simulink model "AWD_Test_ABS_PID"  (Simulink 7.7)
settings: Solver=ode3  StartTime=0.0  StopTime=10  FixedStep=0.001  RelTol=1e-3
undefined symbols (not defined in the file): Bx, By, Cx, Cy, dfilt, Dx, Dy, Ex, Ey, fdesignblkfcn, g, gcbh, hg, Jw, Jz, Lf, Lr, Lw, m, r0, Rw, rx1, rx2, ry1, ry2, T_Avail, Vx0, Vy0, wRL0
libraries: simulink x6, fuzblock x5, dsparch4 x1
settings Model: Creator=ETLAB  LastModifiedBy=Kenny Schmutz
settings DebuggingCC: InheritedTsInSrcMsg=none  FcnCallInpInsideContextMsg=Enable All

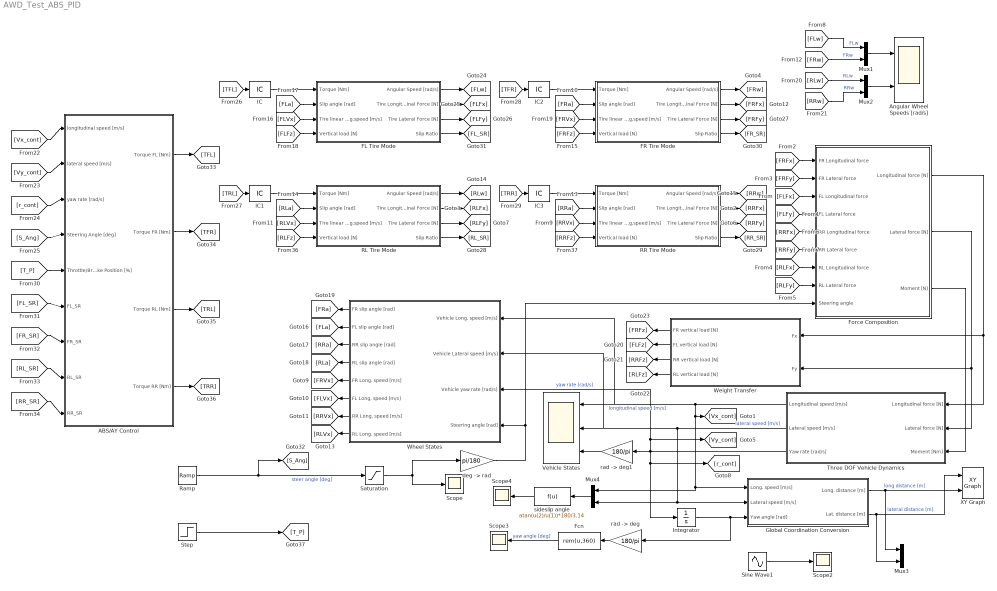
== system AWD_Test_ABS_PID ==
  ABS/AY Control : Subsystem
  Angular Wheel Speeds [rad/s] : Scope  NumInputPorts=2
      settings: YMin=-110~-110  YMax=30~30  SaveName=ScopeData7
  FL Tire Mode : Subsystem
      mask Display:
      | image(imread('Tire.bmp'),'center')
      | port_label('input', 1, 'Torque [Nm]')
      | port_label('input', 2, 'Slip angle [rad]')
      | port_label('input', 3, 'Long. speed [m/s]')
      | port_label('input', 4, 'Vertical load [N]')
      | port_label('output', 1, 'Angular speed [rad/s]')
      | port_label('output', 2, 'Long. force [N]')
      | port_label('output', 3, 'Lateral force [N]')
      | port_label('output', 4, 'Slip Ratio')
  FR Tire Mode : Subsystem
      mask Display:
      | image(imread('Tire.bmp'),'center')
      | port_label('input', 1, 'Torque [Nm]')
      | port_label('input', 2, 'Slip angle [rad]')
      | port_label('input', 3, 'Long. speed [m/s]')
      | port_label('input', 4, 'Vertical load [N]')
      | port_label('output', 1, 'Angular speed [rad/s]')
      | port_label('output', 2, 'Long. force [N]')
      | port_label('output', 3, 'Lateral force [N]')
      | port_label('output', 4, 'Slip Ratio')
  Fcn : Fcn  Expr=rem(u,360)
  Force Composition : Subsystem
  Global Coordination Conversion : Subsystem
  IC{,1..3} (4 alike) : InitialCondition  Value=0
  Integrator : Integrator
  Mux{1..4} (4 alike) : Mux  Inputs=2
  RL Tire Mode : Subsystem
      mask Display:
      | image(imread('Tire.bmp'),'center')
      | port_label('input', 1, 'Torque [Nm]')
      | port_label('input', 2, 'Slip angle [rad]')
      | port_label('input', 3, 'Long. speed [m/s]')
      | port_label('input', 4, 'Vertical load [N]')
      | port_label('output', 1, 'Angular speed [rad/s]')
      | port_label('output', 2, 'Long. force [N]')
      | port_label('output', 3, 'Lateral force [N]')
      | port_label('output', 4, 'Slip Ratio')
  RR Tire Mode : Subsystem
      mask Display:
      | image(imread('Tire.bmp'),'center')
      | port_label('input', 1, 'Torque [Nm]')
      | port_label('input', 2, 'Slip angle [rad]')
      | port_label('input', 3, 'Long. speed [m/s]')
      | port_label('input', 4, 'Vertical load [N]')
      | port_label('output', 1, 'Angular speed [rad/s]')
      | port_label('output', 2, 'Long. force [N]')
      | port_label('output', 3, 'Lateral force [N]')
  Ramp : simulink/Sources/Ramp  SystemSampleTime=-1  slope=0  start=0  X0=0
  Saturation : Saturate  UpperLimit=10  LowerLimit=-10
  Scope{,2..4} (4 alike) : Scope
      Scope settings: YMin=0.93  YMax=1
      Scope2 settings: YMin=0.525  YMax=0.825  SaveName=ScopeData3
      Scope3 settings: SaveName=ScopeData5
      Scope4 settings: YMin=0.0025  YMax=0.05  SaveName=ScopeData20
  Sine Wave1 : Sin  Frequency=0.5  SampleTime=0
  Step : Step  Time=.5  SampleTime=0
  Three DOF Vehicle Dynamics : Subsystem
      mask Display:
      | image(imread('Vehicle.bmp'),'center')
      | port_label('input', 1, 'Longitudinal force [N]')
      | port_label('input', 2, 'Lateral force [N]')
      | port_label('input', 3, 'Moment [Nm]')
      | port_label('output', 1, 'Longitudinal speed [m/s]')
      | port_label('output', 2, 'Lateral speed [m/s]')
      | port_label('output', 3, 'Yaw rate [rad/s]')
  Vehicle States : Scope  NumInputPorts=3
      settings: TimeRange=10  YMin=19.45~3.5e-033~-8.5e-032  YMax=19.56~4.4e-033~-1.5e-032  SaveName=StatesOutpus1
  Weight Transfer : Subsystem
  Wheel States : Subsystem
  XY Graph : simulink/Sinks/XY Graph  SystemSampleTime=-1  xmin=-500  xmax=500  ymin=-500  ymax=500  st=-1
  "deg -> rad" : Gain  Gain=pi/180
  "rad -> deg" : Gain  Gain=180/pi
  "rad -> deg1" : Gain  Gain=180/pi
  sideslip angle : Fcn  Expr=atan(u(2)/u(1))*180/3.14
  wires:
  RL Tire Mode/2(Tire Longitudinal Force [N]) -> [RLFx]
  RL Tire Mode/1(Angular Speed [rad/s]) -> [RLw]
  [RLVx] -> RL Tire Mode/3(Tire linear Long.speed [m/s])
  Wheel States/5(FR Long. speed [m/s]) -> [FRVx]
  Wheel States/6(FL Long. speed [m/s]) -> [FLVx]
  Wheel States/7(RR Long. speed [m/s]) -> [RRVx]
  Wheel States/8(RL Long. speed [m/s]) -> [RLVx]
  Three DOF Vehicle Dynamics/3(Yaw rate [rad/s]) -> "rad -> deg1"/1, Wheel States/3(Vehicle yaw rate [rad/s]), [Vy_cont], Integrator/1, [r_cont]  "yaw rate [rad/s]"
  Three DOF Vehicle Dynamics/2(Lateral speed [m/s]) -> Wheel States/2(Vehicle Lateral speed [m/s]), Global Coordination Conversion/2(Lateral speed [m/s]), Mux4/2, Vehicle States/2  "lateral speed [m/s]"
  Three DOF Vehicle Dynamics/1(Longitudinal speed [m/s]) -> Wheel States/1(Vehicle Long. speed [m/s]), Vehicle States/1, Global Coordination Conversion/1(Long. speed [m/s]), Mux4/1, [Vx_cont]  "longitudinal speed [m/s]"
  Wheel States/1("FR slip angle [rad] ") -> [FRa]
  Wheel States/2("FL slip angle [rad] ") -> [FLa]
  Wheel States/3("RR slip angle [rad] ") -> [RRa]
  Wheel States/4("RL slip angle [rad] ") -> [RLa]
  [RLa] -> RL Tire Mode/2(Slip angle [rad])
  Force Composition/1(Longitudinal force [N]) -> Weight Transfer/1(Fx), Three DOF Vehicle Dynamics/1(Longitudinal force [N])
  [FRFx] -> Force Composition/1(FR Longitudinal force)
  [FRFy] -> Force Composition/2(FR Lateral force)
  [FLFx] -> Force Composition/3(FL Longitudinal force)
  [FLFy] -> Force Composition/4(FL Lateral force)
  [RRFx] -> Force Composition/5(RR Longitudinal force)
  [RRFy] -> Force Composition/6(RR Lateral force)
  [RLFx] -> Force Composition/7(RL Longitudinal force)
  [RLFy] -> Force Composition/8(RL Lateral force)
  "deg -> rad"/1 -> Wheel States/4(Steering angle [rad]), Force Composition/9(Steering angle)
  "rad -> deg"/1 -> Fcn/1
  Fcn/1 -> Scope3/1  "yaw angle [deg]"
  Global Coordination Conversion/1(Long. distance [m]) -> XY Graph/2, Mux3/1  "long distance [m]"
  Global Coordination Conversion/2(Lat. distance [m]) -> XY Graph/1, Mux3/2  "lateral distance [m]"
  Weight Transfer/1(FR vertical load [N]) -> [FRFz]
  Weight Transfer/2(FL vertical load [N]) -> [FLFz]
  Weight Transfer/3(RR vertical load [N]) -> [RRFz]
  Weight Transfer/4(RL vertical load [N]) -> [RLFz]
  [RLFz] -> RL Tire Mode/4(Vertical load [N])
  Force Composition/2(Lateral force [N]) -> Weight Transfer/2(Fy), Three DOF Vehicle Dynamics/2(Lateral force [N])
  Integrator/1 -> Global Coordination Conversion/3(Yaw angle [rad]), "rad -> deg"/1
  RL Tire Mode/3(Tire Lateral Force [N]) -> [RLFy]
  [RRa] -> RR Tire Mode/2(Slip angle [rad])
  [RRVx] -> RR Tire Mode/3(Tire linear Long.speed [m/s])
  [RRFz] -> RR Tire Mode/4(Vertical load [N])
  RR Tire Mode/1(Angular Speed [rad/s]) -> [RRw]
  RR Tire Mode/2(Tire Longitudinal Force [N]) -> [RRFx]
  RR Tire Mode/3(Tire Lateral Force [N]) -> [RRFy]
  Force Composition/3(Moment [N]) -> Three DOF Vehicle Dynamics/3(Moment [Nm])
  "rad -> deg1"/1 -> Vehicle States/3
  Mux4/1 -> sideslip angle/1
  sideslip angle/1 -> Scope4/1
  Ramp/1 -> Saturation/1, [S_Ang]  "steer angle [deg]"
  Sine Wave1/1 -> Scope2/1
  FL Tire Mode/2(Tire Longitudinal Force [N]) -> [FLFx]
  FL Tire Mode/1(Angular Speed [rad/s]) -> [FLw]
  [FLVx] -> FL Tire Mode/3(Tire linear Long.speed [m/s])
  IC/1 -> FL Tire Mode/1(Torque [Nm])
  [FLa] -> FL Tire Mode/2(Slip angle [rad])
  [FLFz] -> FL Tire Mode/4(Vertical load [N])
  FL Tire Mode/3(Tire Lateral Force [N]) -> [FLFy]
  [FRa] -> FR Tire Mode/2(Slip angle [rad])
  [FRVx] -> FR Tire Mode/3(Tire linear Long.speed [m/s])
  [FRFz] -> FR Tire Mode/4(Vertical load [N])
  FR Tire Mode/1(Angular Speed [rad/s]) -> [FRw]
  FR Tire Mode/2(Tire Longitudinal Force [N]) -> [FRFx]
  FR Tire Mode/3(Tire Lateral Force [N]) -> [FRFy]
  Saturation/1 -> "deg -> rad"/1, Scope/1
  [FLw] -> Mux1/1  "FLw"
  [FRw] -> Mux1/2  "FRw"
  [RLw] -> Mux2/1  "RLw"
  [RRw] -> Mux2/2  "RRw"
  Mux1/1 -> Angular Wheel Speeds [rad/s]/1
  Mux2/1 -> Angular Wheel Speeds [rad/s]/2
  [Vx_cont] -> ABS/AY Control/1(longitudinal speed [m/s])
  [Vy_cont] -> ABS/AY Control/2(lateral speed [m/s])
  [r_cont] -> ABS/AY Control/3(yaw rate [rad/s])
  RL Tire Mode/4("Slip Ratio ") -> [RL_SR]
  RR Tire Mode/4(Slip Ratio) -> [RR_SR]
  FR Tire Mode/4(Slip Ratio) -> [FR_SR]
  FL Tire Mode/4(Slip Ratio) -> [FL_SR]
  [S_Ang] -> ABS/AY Control/4(Steering Angle [deg])
  [TFL] -> IC/1
  IC1/1 -> RL Tire Mode/1(Torque [Nm])
  [TRL] -> IC1/1
  IC2/1 -> FR Tire Mode/1(Torque [Nm])
  [TFR] -> IC2/1
  IC3/1 -> RR Tire Mode/1(Torque [Nm])
  [TRR] -> IC3/1
  ABS/AY Control/1(Torque FL [Nm]) -> [TFL]
  ABS/AY Control/2(Torque FR [Nm]) -> [TFR]
  ABS/AY Control/3(Torque RL [Nm]) -> [TRL]
  ABS/AY Control/4(Torque RR [Nm]) -> [TRR]
  [T_P] -> ABS/AY Control/5(Throttle/Brake Position [%])
  [FL_SR] -> ABS/AY Control/6(FL_SR)
  [FR_SR] -> ABS/AY Control/7(FR_SR)
  [RL_SR] -> ABS/AY Control/8(RL_SR)
  [RR_SR] -> ABS/AY Control/9(RR_SR)
  Step/1 -> [T_P]

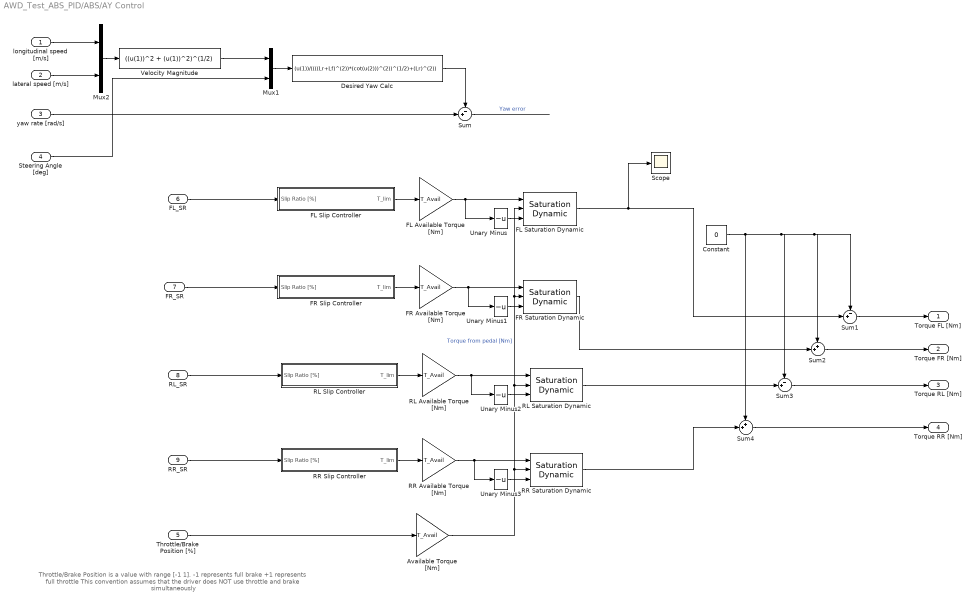
== system AWD_Test_ABS_PID/ABS/AY Control ==
  note: Throttle/Brake Position is a value with range [-1 1].
      | -1 represents full brake
      | +1 represents full throttle
      | This convention assumes that the driver does NOT use throttle and brake simultaneously
  longitudinal speed [m/s] : Inport
  lateral speed [m/s] : Inport  Port=2
  yaw rate [rad/s] : Inport  Port=3
  Steering Angle [deg] : Inport  Port=4
  Throttle/Brake Position [%] : Inport  Port=5
  FL_SR : Inport  Port=6
  FR_SR : Inport  Port=7
  RL_SR : Inport  Port=8
  RR_SR : Inport  Port=9
  Available Torque [Nm] : Gain  Gain=T_Avail
  Constant : Constant  Value=0
  Desired Yaw Calc : Fcn  Expr=(u(1))/((((Lr+Lf)^(2))*(cot(u(2)))^(2))^(1/2)+(Lr)^(2))
  FL Available Torque [Nm] : Gain  Gain=T_Avail
  FL Saturation Dynamic : simulink/Discontinuities/Saturation Dynamic  SystemSampleTime=-1  OutMin=[]  OutMax=[]  OutDataTypeStr=Inherit: Same as second input  OutDataType=fixdt(1, 16)  OutScaling=2^-10  DoSatur=off
  FL Slip Controller : Subsystem
  FR Available Torque [Nm] : Gain  Gain=T_Avail
  FR Saturation Dynamic : simulink/Discontinuities/Saturation Dynamic  SystemSampleTime=-1  OutMin=[]  OutMax=[]  OutDataTypeStr=Inherit: Same as second input  OutDataType=fixdt(1, 16)  OutScaling=2^-10  DoSatur=off
  FR Slip Controller : Subsystem
  Mux1 : Mux  Inputs=2
  Mux2 : Mux  Inputs=2
  RL Available Torque [Nm] : Gain  Gain=T_Avail
  RL Saturation Dynamic : simulink/Discontinuities/Saturation Dynamic  SystemSampleTime=-1  OutMin=[]  OutMax=[]  OutDataTypeStr=Inherit: Same as second input  OutDataType=fixdt(1, 16)  OutScaling=2^-10  DoSatur=off
  RL Slip Controller : Subsystem
  RR Available Torque [Nm] : Gain  Gain=T_Avail
  RR Saturation Dynamic : simulink/Discontinuities/Saturation Dynamic  SystemSampleTime=-1  OutMin=[]  OutMax=[]  OutDataTypeStr=Inherit: Same as second input  OutDataType=fixdt(1, 16)  OutScaling=2^-10  DoSatur=off
  RR Slip Controller : Subsystem
  Scope : Scope
      settings: YMin=-93.5444  YMax=-84.6354  SaveName=ScopeData9
  Sum : Sum  Inputs=-+|
  Sum1 : Sum  Inputs=-+|
  Sum2 : Sum  Inputs=++|
  Sum3 : Sum  Inputs=-+|
  Sum4 : Sum  Inputs=++|
  Unary Minus{,1..3} (4 alike) : UnaryMinus
  Velocity Magnitude : Fcn  Expr=((u(1))^2 + (u(1))^2)^(1/2)
  Torque FL [Nm] : Outport
  Torque FR [Nm] : Outport  Port=2
  Torque RL [Nm] : Outport  Port=3
  Torque RR [Nm] : Outport  Port=4
  wires:
  Mux1/1 -> Desired Yaw Calc/1
  lateral speed [m/s]/1 -> Mux2/2
  longitudinal speed [m/s]/1 -> Mux2/1
  Mux2/1 -> Velocity Magnitude/1
  Velocity Magnitude/1 -> Mux1/1
  Steering Angle [deg]/1 -> Mux1/2
  yaw rate [rad/s]/1 -> Sum/2
  Desired Yaw Calc/1 -> Sum/1
  Sum/1 -> ?  "Yaw error"
  Sum1/1 -> Torque FL [Nm]/1
  Sum2/1 -> Torque FR [Nm]/1
  Sum3/1 -> Torque RL [Nm]/1
  Sum4/1 -> Torque RR [Nm]/1
  Throttle/Brake Position [%]/1 -> Available Torque [Nm]/1
  Available Torque [Nm]/1 -> RR Saturation Dynamic/2, RL Saturation Dynamic/2, FR Saturation Dynamic/2, FL Saturation Dynamic/2  "Torque from pedal [Nm]"
  FL_SR/1 -> FL Slip Controller/1(Slip Ratio [%])
  FR_SR/1 -> FR Slip Controller/1(Slip Ratio [%])
  RL_SR/1 -> RL Slip Controller/1(Slip Ratio [%])
  RR_SR/1 -> RR Slip Controller/1(Slip Ratio [%])
  FL Slip Controller/1(T_lim) -> FL Available Torque [Nm]/1
  FR Slip Controller/1(T_lim) -> FR Available Torque [Nm]/1
  RL Slip Controller/1(T_lim) -> RL Available Torque [Nm]/1
  RR Slip Controller/1(T_lim) -> RR Available Torque [Nm]/1
  FL Available Torque [Nm]/1 -> FL Saturation Dynamic/1, Unary Minus/1
  Unary Minus/1 -> FL Saturation Dynamic/3
  FR Available Torque [Nm]/1 -> FR Saturation Dynamic/1, Unary Minus1/1
  Unary Minus1/1 -> FR Saturation Dynamic/3
  RL Available Torque [Nm]/1 -> RL Saturation Dynamic/1, Unary Minus2/1
  RR Available Torque [Nm]/1 -> RR Saturation Dynamic/1, Unary Minus3/1
  Unary Minus2/1 -> RL Saturation Dynamic/3
  Unary Minus3/1 -> RR Saturation Dynamic/3
  RR Saturation Dynamic/1 -> Sum4/2
  RL Saturation Dynamic/1 -> Sum3/2
  FR Saturation Dynamic/1 -> Sum2/2
  FL Saturation Dynamic/1 -> Sum1/2, Scope/1
  Constant/1 -> Sum4/1, Sum3/1, Sum1/1, Sum2/1

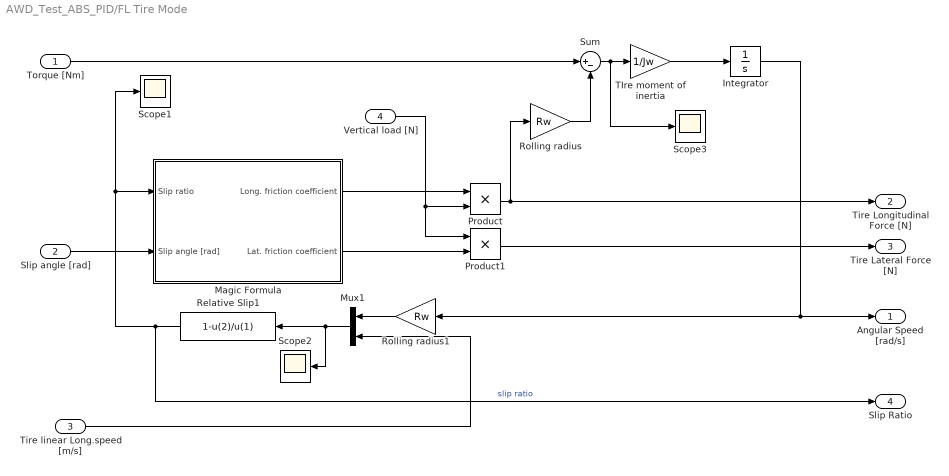
== system AWD_Test_ABS_PID/FL Tire Mode ==
  Torque [Nm] : Inport
  Slip angle [rad] : Inport  Port=2
  Tire linear Long.speed [m/s] : Inport  Port=3
  Vertical load [N] : Inport  Port=4
  Integrator : Integrator  InitialCondition=wRL0
  Magic Formula : Subsystem
      mask Type: Magic Formula (Combined Slip)
      mask Display:
      | image(imread('Magic formula.jpg'),'center')
      | port_label('input', 1, 'slip ratio')
      | port_label('input', 2, 'slip angle')
      | port_label('output', 1, 'Mux')
      | port_label('output', 2, 'Muy')
  Mux1 : Mux  Inputs=2
  Product : Product  RndMeth=Zero
  Product1 : Product  RndMeth=Zero
  Relative Slip1 : Fcn  Expr=1-u(2)/u(1)
  Rolling radius : Gain  Gain=Rw  SaturateOnIntegerOverflow=on  OutDataTypeStr=Inherit: Same as input  ParamDataTypeStr=Inherit: Same as input
  Rolling radius1 : Gain  Gain=Rw  SaturateOnIntegerOverflow=on  OutDataTypeStr=Inherit: Same as input  ParamDataTypeStr=Inherit: Same as input
  Scope1 : Scope
      settings: YMin=0.0014905  YMax=0.0014955  SaveName=ScopeData2
  Scope2 : Scope
      settings: YMin=0.001  YMax=0.013  SaveName=ScopeData11
  Scope3 : Scope
      settings: YMin=-9.46434  YMax=-9.46434  SaveName=ScopeData14
  Sum : Sum  Inputs=|+-
  TIre moment of inertia : Gain  Gain=1/Jw  SaturateOnIntegerOverflow=on  OutDataTypeStr=Inherit: Same as input  ParamDataTypeStr=Inherit: Same as input
  Angular Speed [rad/s] : Outport
  Tire Longitudinal Force [N] : Outport  Port=2
  Tire Lateral Force [N] : Outport  Port=3
  Slip Ratio : Outport  Port=4
  wires:
  Slip angle [rad]/1 -> Magic Formula/2(Slip angle [rad])
  Relative Slip1/1 -> Magic Formula/1(Slip ratio), Scope1/1, Slip Ratio/1  "slip ratio"
  Tire linear Long.speed [m/s]/1 -> Mux1/2
  Torque [Nm]/1 -> Sum/1
  Sum/1 -> TIre moment of inertia/1, Scope3/1
  TIre moment of inertia/1 -> Integrator/1
  Integrator/1 -> Angular Speed [rad/s]/1, Rolling radius1/1
  Rolling radius/1 -> Sum/2
  Mux1/1 -> Relative Slip1/1, Scope2/1
  Rolling radius1/1 -> Mux1/1
  Magic Formula/1(Long. friction coefficient) -> Product/1
  Magic Formula/2(Lat. friction coefficient) -> Product1/2
  Product/1 -> Rolling radius/1, Tire Longitudinal Force [N]/1
  Vertical load [N]/1 -> Product/2, Product1/1
  Product1/1 -> Tire Lateral Force [N]/1

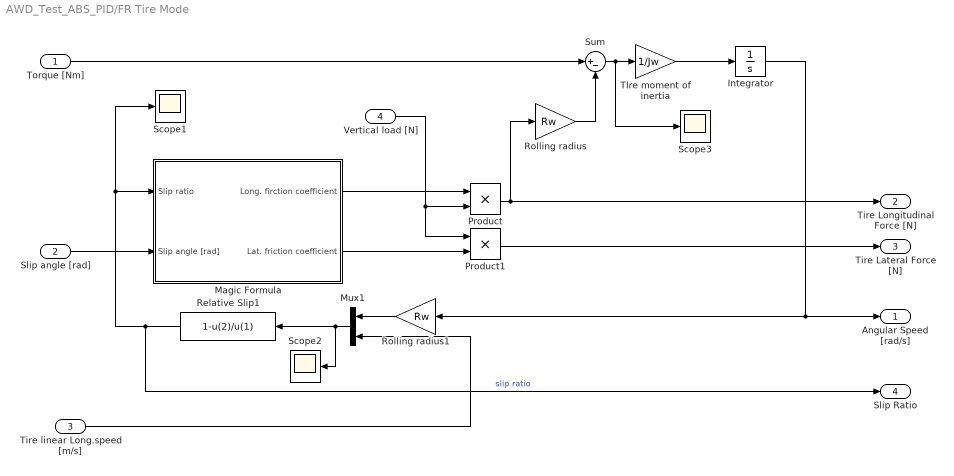
== system AWD_Test_ABS_PID/FR Tire Mode ==
  Torque [Nm] : Inport
  Slip angle [rad] : Inport  Port=2
  Tire linear Long.speed [m/s] : Inport  Port=3
  Vertical load [N] : Inport  Port=4
  Integrator : Integrator  InitialCondition=wRL0
  Magic Formula : Subsystem
      mask Type: Magic Formula (Combined Slip)
      mask Display:
      | image(imread('Magic formula.jpg'),'center')
      | port_label('input', 1, 'slip ratio')
      | port_label('input', 2, 'slip angle')
      | port_label('output', 1, 'Mux')
      | port_label('output', 2, 'Muy')
  Mux1 : Mux  Inputs=2
  Product : Product  RndMeth=Zero
  Product1 : Product  RndMeth=Zero
  Relative Slip1 : Fcn  Expr=1-u(2)/u(1)
  Rolling radius : Gain  Gain=Rw  SaturateOnIntegerOverflow=on  OutDataTypeStr=Inherit: Same as input  ParamDataTypeStr=Inherit: Same as input
  Rolling radius1 : Gain  Gain=Rw  SaturateOnIntegerOverflow=on  OutDataTypeStr=Inherit: Same as input  ParamDataTypeStr=Inherit: Same as input
  Scope1 : Scope
      settings: YMin=0.0014905  YMax=0.0014955  SaveName=ScopeData2
  Scope2 : Scope
      settings: YMin=0.001  YMax=0.013  SaveName=ScopeData11
  Scope3 : Scope
      settings: SaveName=ScopeData14
  Sum : Sum  Inputs=|+-
  TIre moment of inertia : Gain  Gain=1/Jw  SaturateOnIntegerOverflow=on  OutDataTypeStr=Inherit: Same as input  ParamDataTypeStr=Inherit: Same as input
  Angular Speed [rad/s] : Outport
  Tire Longitudinal Force [N] : Outport  Port=2
  Tire Lateral Force [N] : Outport  Port=3
  Slip Ratio : Outport  Port=4
  wires:
  Product1/1 -> Tire Lateral Force [N]/1
  Vertical load [N]/1 -> Product1/1, Product/2
  Product/1 -> Tire Longitudinal Force [N]/1, Rolling radius/1
  Magic Formula/2(Lat. friction coefficient) -> Product1/2
  Magic Formula/1(Long. firction coefficient) -> Product/1
  Rolling radius1/1 -> Mux1/1
  Mux1/1 -> Relative Slip1/1, Scope2/1
  Rolling radius/1 -> Sum/2
  Integrator/1 -> Rolling radius1/1, Angular Speed [rad/s]/1
  TIre moment of inertia/1 -> Integrator/1
  Sum/1 -> Scope3/1, TIre moment of inertia/1
  Torque [Nm]/1 -> Sum/1
  Tire linear Long.speed [m/s]/1 -> Mux1/2
  Relative Slip1/1 -> Scope1/1, Magic Formula/1(Slip ratio), Slip Ratio/1  "slip ratio"
  Slip angle [rad]/1 -> Magic Formula/2(Slip angle [rad])

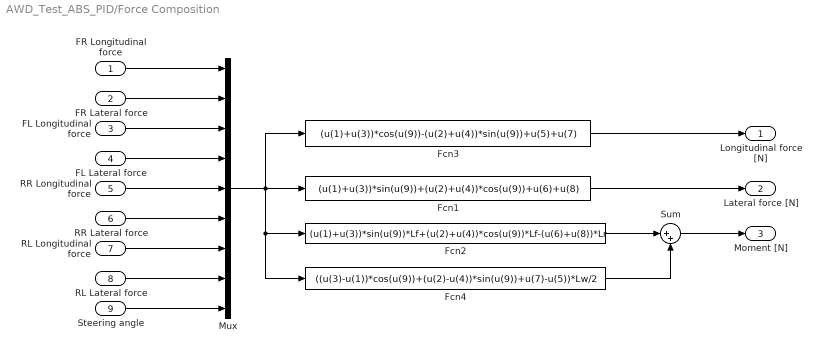
== system AWD_Test_ABS_PID/Force Composition ==
  FR Longitudinal force : Inport
  FR Lateral force : Inport  Port=2
  FL Longitudinal force : Inport  Port=3
  FL Lateral force : Inport  Port=4
  RR Longitudinal force : Inport  Port=5
  RR Lateral force : Inport  Port=6
  RL Longitudinal force : Inport  Port=7
  RL Lateral force : Inport  Port=8
  Steering angle : Inport  Port=9
  Fcn1 : Fcn  Expr=(u(1)+u(3))*sin(u(9))+(u(2)+u(4))*cos(u(9))+u(6)+u(8)
  Fcn2 : Fcn  Expr=(u(1)+u(3))*sin(u(9))*Lf+(u(2)+u(4))*cos(u(9))*Lf-(u(6)+u(8))*Lr
  Fcn3 : Fcn  Expr=(u(1)+u(3))*cos(u(9))-(u(2)+u(4))*sin(u(9))+u(5)+u(7)
  Fcn4 : Fcn  Expr=((u(3)-u(1))*cos(u(9))+(u(2)-u(4))*sin(u(9))+u(7)-u(5))*Lw/2
  Mux : Mux  Inputs=9
  Sum : Sum  Inputs=|++
  Longitudinal force [N] : Outport
  Lateral force [N] : Outport  Port=2
  Moment [N] : Outport  Port=3
  wires:
  Mux/1 -> Fcn3/1, Fcn1/1, Fcn2/1, Fcn4/1
  Fcn3/1 -> Longitudinal force [N]/1
  Fcn1/1 -> Lateral force [N]/1
  Sum/1 -> Moment [N]/1
  Fcn2/1 -> Sum/1
  Fcn4/1 -> Sum/2
  FR Longitudinal force/1 -> Mux/1
  FR Lateral force/1 -> Mux/2
  FL Longitudinal force/1 -> Mux/3
  FL Lateral force/1 -> Mux/4
  RR Longitudinal force/1 -> Mux/5
  RR Lateral force/1 -> Mux/6
  RL Longitudinal force/1 -> Mux/7
  RL Lateral force/1 -> Mux/8
  Steering angle/1 -> Mux/9

== system AWD_Test_ABS_PID/Global Coordination Conversion ==
  Long. speed [m/s] : Inport
  Lateral speed [m/s] : Inport  Port=2
  Yaw angle [rad] : Inport  Port=3
  Fcn : Fcn  Expr=cos(u(3))*u(1)-sin(u(3))*u(2)
  Fcn1 : Fcn  Expr=sin(u(3))*u(1)+cos(u(3))*u(2)
  Integrator : Integrator
  Integrator1 : Integrator
  Mux : Mux  Inputs=3
  Long. distance [m] : Outport
  Lat. distance [m] : Outport  Port=2
  wires:
  Long. speed [m/s]/1 -> Mux/1
  Lateral speed [m/s]/1 -> Mux/2
  Yaw angle [rad]/1 -> Mux/3
  Mux/1 -> Fcn/1, Fcn1/1
  Fcn/1 -> Integrator/1
  Fcn1/1 -> Integrator1/1
  Integrator/1 -> Long. distance [m]/1
  Integrator1/1 -> Lat. distance [m]/1

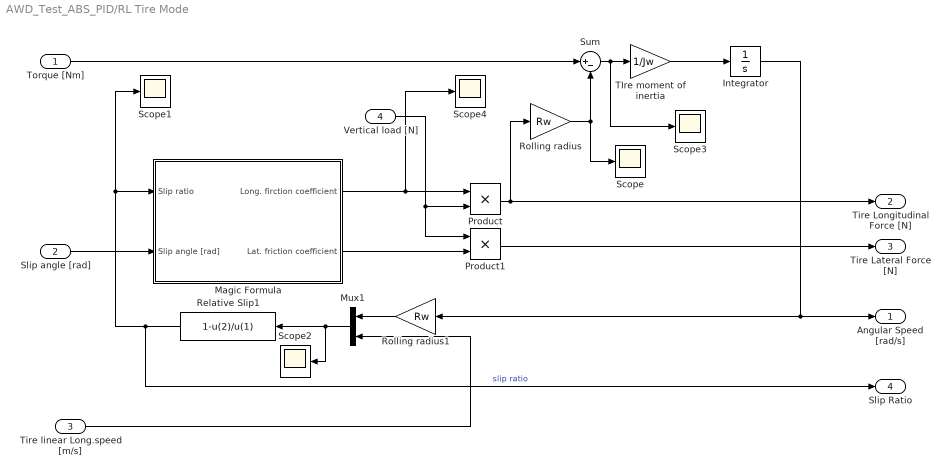
== system AWD_Test_ABS_PID/RL Tire Mode ==
  Torque [Nm] : Inport
  Slip angle [rad] : Inport  Port=2
  Tire linear Long.speed [m/s] : Inport  Port=3
  Vertical load [N] : Inport  Port=4
  Integrator : Integrator  InitialCondition=wRL0
  Magic Formula : Subsystem
      mask Type: Magic Formula (Combined Slip)
      mask Display:
      | image(imread('Magic formula.jpg'),'center')
      | port_label('input', 1, 'slip ratio')
      | port_label('input', 2, 'slip angle')
      | port_label('output', 1, 'Mux')
      | port_label('output', 2, 'Muy')
  Mux1 : Mux  Inputs=2
  Product : Product  RndMeth=Zero
  Product1 : Product  RndMeth=Zero
  Relative Slip1 : Fcn  Expr=1-u(2)/u(1)
  Rolling radius : Gain  Gain=Rw  SaturateOnIntegerOverflow=on  OutDataTypeStr=Inherit: Same as input  ParamDataTypeStr=Inherit: Same as input
  Rolling radius1 : Gain  Gain=Rw  SaturateOnIntegerOverflow=on  OutDataTypeStr=Inherit: Same as input  ParamDataTypeStr=Inherit: Same as input
  Scope{,1..4} (5 alike) : Scope
      Scope settings: SaveName=ScopeData10
      Scope1 settings: YMin=0.0014905  YMax=0.0014955  SaveName=ScopeData2
      Scope2 settings: YMin=0.001  YMax=0.013  SaveName=ScopeData11
      Scope3 settings: SaveName=ScopeData14
      Scope4 settings: SaveName=ScopeData12
  Sum : Sum  Inputs=|+-
  TIre moment of inertia : Gain  Gain=1/Jw  SaturateOnIntegerOverflow=on  OutDataTypeStr=Inherit: Same as input  ParamDataTypeStr=Inherit: Same as input
  Angular Speed [rad/s] : Outport
  Tire Longitudinal Force [N] : Outport  Port=2
  Tire Lateral Force [N] : Outport  Port=3
  "Slip Ratio " : Outport  Port=4
  wires:
  Slip angle [rad]/1 -> Magic Formula/2(Slip angle [rad])
  Relative Slip1/1 -> Magic Formula/1(Slip ratio), Scope1/1, "Slip Ratio "/1  "slip ratio"
  Tire linear Long.speed [m/s]/1 -> Mux1/2
  Torque [Nm]/1 -> Sum/1
  Sum/1 -> TIre moment of inertia/1, Scope3/1
  TIre moment of inertia/1 -> Integrator/1
  Integrator/1 -> Angular Speed [rad/s]/1, Rolling radius1/1
  Rolling radius/1 -> Sum/2, Scope/1
  Mux1/1 -> Relative Slip1/1, Scope2/1
  Rolling radius1/1 -> Mux1/1
  Magic Formula/1(Long. firction coefficient) -> Product/1, Scope4/1
  Magic Formula/2(Lat. friction coefficient) -> Product1/2
  Product/1 -> Rolling radius/1, Tire Longitudinal Force [N]/1
  Vertical load [N]/1 -> Product/2, Product1/1
  Product1/1 -> Tire Lateral Force [N]/1

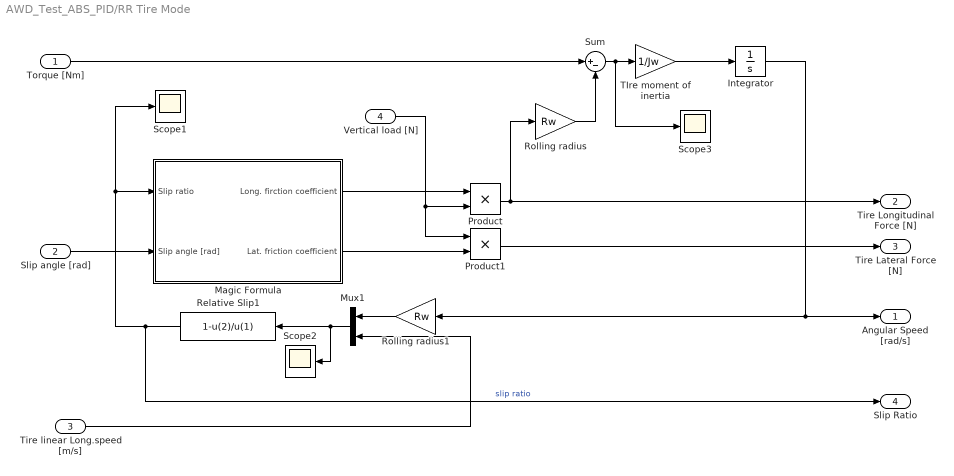
== system AWD_Test_ABS_PID/RR Tire Mode ==
  Torque [Nm] : Inport
  Slip angle [rad] : Inport  Port=2
  Tire linear Long.speed [m/s] : Inport  Port=3
  Vertical load [N] : Inport  Port=4
  Integrator : Integrator  InitialCondition=wRL0
  Magic Formula : Subsystem
      mask Type: Magic Formula (Combined Slip)
      mask Display:
      | image(imread('Magic formula.jpg'),'center')
      | port_label('input', 1, 'slip ratio')
      | port_label('input', 2, 'slip angle')
      | port_label('output', 1, 'Mux')
      | port_label('output', 2, 'Muy')
  Mux1 : Mux  Inputs=2
  Product : Product  RndMeth=Zero
  Product1 : Product  RndMeth=Zero
  Relative Slip1 : Fcn  Expr=1-u(2)/u(1)
  Rolling radius : Gain  Gain=Rw  SaturateOnIntegerOverflow=on  OutDataTypeStr=Inherit: Same as input  ParamDataTypeStr=Inherit: Same as input
  Rolling radius1 : Gain  Gain=Rw  SaturateOnIntegerOverflow=on  OutDataTypeStr=Inherit: Same as input  ParamDataTypeStr=Inherit: Same as input
  Scope1 : Scope
      settings: YMin=0.0014905  YMax=0.0014955  SaveName=ScopeData2
  Scope2 : Scope
      settings: YMin=0.001  YMax=0.013  SaveName=ScopeData11
  Scope3 : Scope
      settings: SaveName=ScopeData14
  Sum : Sum  Inputs=|+-
  TIre moment of inertia : Gain  Gain=1/Jw  SaturateOnIntegerOverflow=on  OutDataTypeStr=Inherit: Same as input  ParamDataTypeStr=Inherit: Same as input
  Angular Speed [rad/s] : Outport
  Tire Longitudinal Force [N] : Outport  Port=2
  Tire Lateral Force [N] : Outport  Port=3
  Slip Ratio : Outport  Port=4
  wires:
  Product1/1 -> Tire Lateral Force [N]/1
  Vertical load [N]/1 -> Product1/1, Product/2
  Product/1 -> Tire Longitudinal Force [N]/1, Rolling radius/1
  Magic Formula/2(Lat. friction coefficient) -> Product1/2
  Magic Formula/1(Long. firction coefficient) -> Product/1
  Rolling radius1/1 -> Mux1/1
  Mux1/1 -> Relative Slip1/1, Scope2/1
  Rolling radius/1 -> Sum/2
  Integrator/1 -> Rolling radius1/1, Angular Speed [rad/s]/1
  TIre moment of inertia/1 -> Integrator/1
  Sum/1 -> Scope3/1, TIre moment of inertia/1
  Torque [Nm]/1 -> Sum/1
  Tire linear Long.speed [m/s]/1 -> Mux1/2
  Relative Slip1/1 -> Scope1/1, Magic Formula/1(Slip ratio), Slip Ratio/1  "slip ratio"
  Slip angle [rad]/1 -> Magic Formula/2(Slip angle [rad])

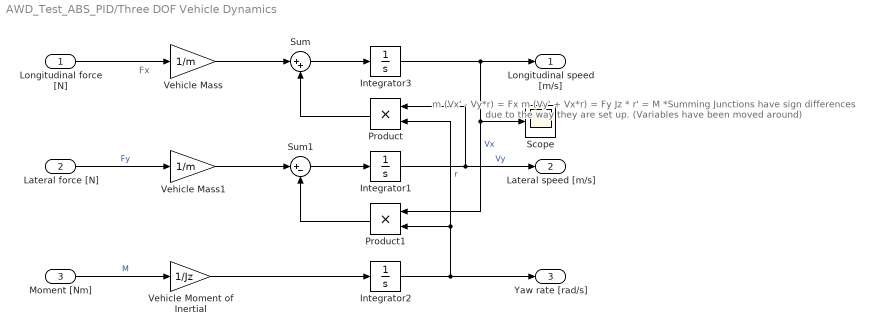
== system AWD_Test_ABS_PID/Three DOF Vehicle Dynamics ==
  note: m (Vx' - Vy*r) = Fx
      | m (Vy' + Vx*r) = Fy
      |
      | Jz * r' = M
      |
      | *Summing Junctions have sign differences due to
      | the way they are set up. (Variables have been moved around)
  note: Fx
  Longitudinal force [N] : Inport
  Lateral force [N] : Inport  Port=2
  Moment [Nm] : Inport  Port=3
  Integrator1 : Integrator  InitialCondition=Vy0  UpperSaturationLimit=1000  LowerSaturationLimit=0
  Integrator2 : Integrator  InitialCondition=r0
  Integrator3 : Integrator  InitialCondition=Vx0  UpperSaturationLimit=1000  LowerSaturationLimit=0
  Product : Product  RndMeth=Zero
  Product1 : Product  RndMeth=Zero
  Scope : Scope
      settings: SaveName=ScopeData18
  Sum : Sum  Inputs=|++
  Sum1 : Sum  Inputs=|+-
  Vehicle Mass : Gain  Gain=1/m
  Vehicle Mass1 : Gain  Gain=1/m
  Vehicle Moment of Inertial : Gain  Gain=1/Jz
  Longitudinal speed [m/s] : Outport
  Lateral speed [m/s] : Outport  Port=2
  Yaw rate [rad/s] : Outport  Port=3
  wires:
  Integrator2/1 -> Yaw rate [rad/s]/1, Product/2, Product1/2  "r"
  Moment [Nm]/1 -> Vehicle Moment of Inertial/1  "M"
  Integrator1/1 -> Product/1, Lateral speed [m/s]/1  "Vy"
  Integrator3/1 -> Longitudinal speed [m/s]/1, Product1/1, Scope/1  "Vx"
  Vehicle Moment of Inertial/1 -> Integrator2/1
  Vehicle Mass1/1 -> Sum1/1
  Lateral force [N]/1 -> Vehicle Mass1/1  "Fy"
  Vehicle Mass/1 -> Sum/1
  Sum1/1 -> Integrator1/1
  Product1/1 -> Sum1/2
  Sum/1 -> Integrator3/1
  Product/1 -> Sum/2
  Longitudinal force [N]/1 -> Vehicle Mass/1

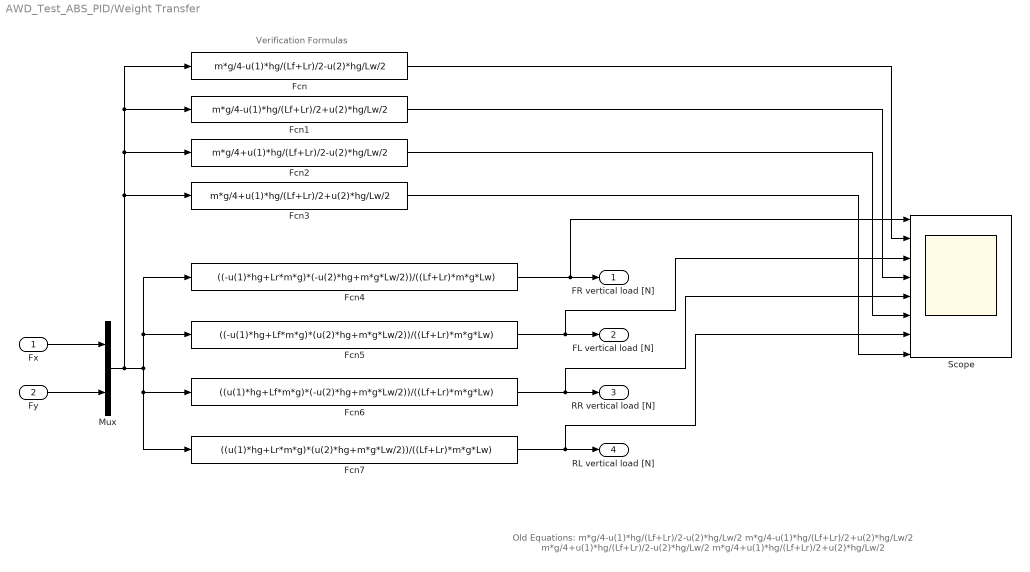
== system AWD_Test_ABS_PID/Weight Transfer ==
  note: Old Equations:
      | m*g/4-u(1)*hg/(Lf+Lr)/2-u(2)*hg/Lw/2
      | m*g/4-u(1)*hg/(Lf+Lr)/2+u(2)*hg/Lw/2
      | m*g/4+u(1)*hg/(Lf+Lr)/2-u(2)*hg/Lw/2
      | m*g/4+u(1)*hg/(Lf+Lr)/2+u(2)*hg/Lw/2
  note: Verification Formulas
  Fx : Inport
  Fy : Inport  Port=2
  Fcn : Fcn  Expr=m*g/4-u(1)*hg/(Lf+Lr)/2-u(2)*hg/Lw/2
  Fcn1 : Fcn  Expr=m*g/4-u(1)*hg/(Lf+Lr)/2+u(2)*hg/Lw/2
  Fcn2 : Fcn  Expr=m*g/4+u(1)*hg/(Lf+Lr)/2-u(2)*hg/Lw/2
  Fcn3 : Fcn  Expr=m*g/4+u(1)*hg/(Lf+Lr)/2+u(2)*hg/Lw/2
  Fcn4 : Fcn  Expr=((-u(1)*hg+Lr*m*g)*(-u(2)*hg+m*g*Lw/2))/((Lf+Lr)*m*g*Lw)
  Fcn5 : Fcn  Expr=((-u(1)*hg+Lf*m*g)*(u(2)*hg+m*g*Lw/2))/((Lf+Lr)*m*g*Lw)
  Fcn6 : Fcn  Expr=((u(1)*hg+Lf*m*g)*(-u(2)*hg+m*g*Lw/2))/((Lf+Lr)*m*g*Lw)
  Fcn7 : Fcn  Expr=((u(1)*hg+Lr*m*g)*(u(2)*hg+m*g*Lw/2))/((Lf+Lr)*m*g*Lw)
  Mux : Mux  Inputs=2
  Scope : Scope  NumInputPorts=8
      settings: TimeRange=20  YMin=0~3100~3800~4000~3100~3100~4000~4000  YMax=10000~3400~4400~4300~3400~3400~4300~4300  SaveName=ScopeData6  MaxDataPoints=21000
  FR vertical load [N] : Outport
  FL vertical load [N] : Outport  Port=2
  RR vertical load [N] : Outport  Port=3
  RL vertical load [N] : Outport  Port=4
  wires:
  Fy/1 -> Mux/2
  Fx/1 -> Mux/1
  Fcn4/1 -> FR vertical load [N]/1, Scope/1
  Fcn5/1 -> FL vertical load [N]/1, Scope/3
  Fcn6/1 -> RR vertical load [N]/1, Scope/5
  Fcn7/1 -> RL vertical load [N]/1, Scope/7
  Fcn/1 -> Scope/2
  Fcn1/1 -> Scope/4
  Fcn2/1 -> Scope/6
  Fcn3/1 -> Scope/8
  Mux/1 -> Fcn4/1, Fcn5/1, Fcn6/1, Fcn7/1, Fcn3/1, Fcn2/1, Fcn1/1, Fcn/1

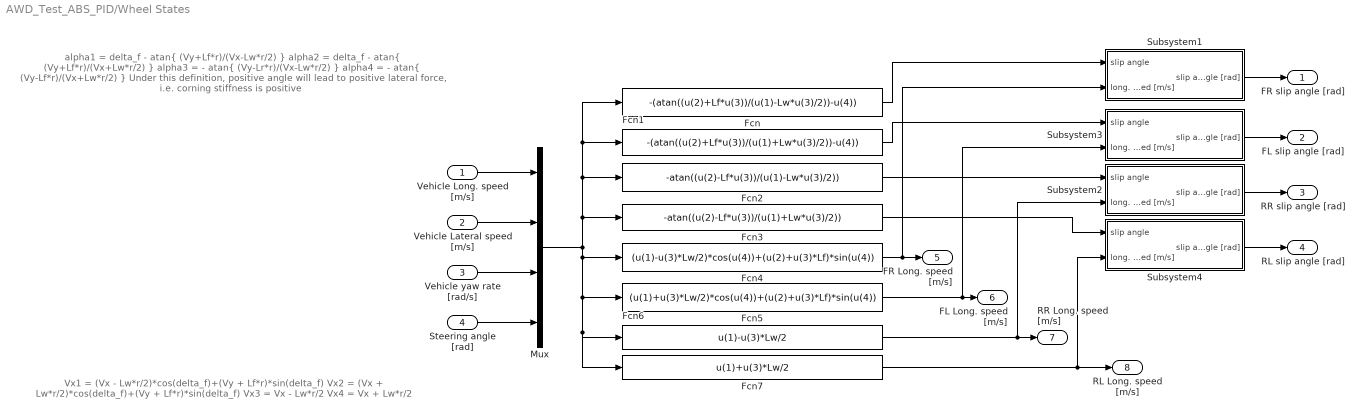
== system AWD_Test_ABS_PID/Wheel States ==
  note: alpha1 = delta_f - atan{ (Vy+Lf*r)/(Vx-Lw*r/2) }
      | alpha2 = delta_f - atan{ (Vy+Lf*r)/(Vx+Lw*r/2) }
      | alpha3 = - atan{ (Vy-Lr*r)/(Vx-Lw*r/2) }
      | alpha4 = - atan{ (Vy-Lf*r)/(Vx+Lw*r/2) }
      | Under this definition, positive angle will lead to  positive lateral force,
      | i.e. corning stiffness is positive
  note: Vx1 = (Vx - Lw*r/2)*cos(delta_f)+(Vy + Lf*r)*sin(delta_f)
      | Vx2 = (Vx + Lw*r/2)*cos(delta_f)+(Vy + Lf*r)*sin(delta_f)
      | Vx3 = Vx - Lw*r/2
      | Vx4 = Vx + Lw*r/2
  Vehicle Long. speed [m/s] : Inport
  Vehicle Lateral speed [m/s] : Inport  Port=2
  Vehicle yaw rate [rad/s] : Inport  Port=3
  Steering angle [rad] : Inport  Port=4
  Fcn : Fcn  Expr=-(atan((u(2)+Lf*u(3))/(u(1)-Lw*u(3)/2))-u(4))
  Fcn1 : Fcn  Expr=-(atan((u(2)+Lf*u(3))/(u(1)+Lw*u(3)/2))-u(4))
  Fcn2 : Fcn  Expr=-atan((u(2)-Lf*u(3))/(u(1)-Lw*u(3)/2))
  Fcn3 : Fcn  Expr=-atan((u(2)-Lf*u(3))/(u(1)+Lw*u(3)/2))
  Fcn4 : Fcn  Expr=(u(1)-u(3)*Lw/2)*cos(u(4))+(u(2)+u(3)*Lf)*sin(u(4))
  Fcn5 : Fcn  Expr=(u(1)+u(3)*Lw/2)*cos(u(4))+(u(2)+u(3)*Lf)*sin(u(4))
  Fcn6 : Fcn  Expr=u(1)-u(3)*Lw/2
  Fcn7 : Fcn  Expr=u(1)+u(3)*Lw/2
  Mux : Mux
  Subsystem1 : Subsystem
  Subsystem2 : Subsystem
  Subsystem3 : Subsystem
  Subsystem4 : Subsystem
  "FR slip angle [rad] " : Outport
  "FL slip angle [rad] " : Outport  Port=2
  "RR slip angle [rad] " : Outport  Port=3
  "RL slip angle [rad] " : Outport  Port=4
  FR Long. speed [m/s] : Outport  Port=5
  FL Long. speed [m/s] : Outport  Port=6
  RR Long. speed [m/s] : Outport  Port=7
  RL Long. speed [m/s] : Outport  Port=8
  wires:
  Vehicle yaw rate [rad/s]/1 -> Mux/3
  Vehicle Lateral speed [m/s]/1 -> Mux/2
  Vehicle Long. speed [m/s]/1 -> Mux/1
  Steering angle [rad]/1 -> Mux/4
  Fcn4/1 -> FR Long. speed [m/s]/1, Subsystem1/2(long. speed [m/s])
  Fcn5/1 -> FL Long. speed [m/s]/1, Subsystem3/2(long. speed [m/s])
  Fcn6/1 -> RR Long. speed [m/s]/1, Subsystem2/2(long. speed [m/s])
  Fcn7/1 -> RL Long. speed [m/s]/1, Subsystem4/2(long. speed [m/s])
  Mux/1 -> Fcn5/1, Fcn7/1, Fcn6/1, Fcn4/1, Fcn3/1, Fcn2/1, Fcn1/1, Fcn/1
  Subsystem1/1(slip angle [rad]) -> "FR slip angle [rad] "/1
  Fcn/1 -> Subsystem1/1(slip angle)
  Subsystem3/1(slip angle [rad]) -> "FL slip angle [rad] "/1
  Fcn1/1 -> Subsystem3/1(slip angle)
  Fcn2/1 -> Subsystem2/1(slip angle)
  Fcn3/1 -> Subsystem4/1(slip angle)
  Subsystem2/1(slip angle [rad]) -> "RR slip angle [rad] "/1
  Subsystem4/1(slip angle [rad]) -> "RL slip angle [rad] "/1

== system AWD_Test_ABS_PID/ABS/AY Control/FL Slip Controller ==
  Slip Ratio [%] : Inport
  Abs : Abs
  Derivative : Derivative
  Fuzzy Logic  Controller  with Ruleviewer : fuzblock/Fuzzy Logic  Controller  with Ruleviewer  SystemSampleTime=-1  fismatrix=Fuzzy_Slip_Controller  Ts=.1
  Lowpass Filter : Subsystem  DialogController=fdesignblkfcn  DialogControllerArgs=DataTag1  InitFcn=fdesignblkfcn(gcbh, {'InitFcn'});
      settings: CopyFcn=fdesignblkfcn(gcbh, {'CopyFcn'});
      mask Type: Lowpass Filter
      mask Description: Design a lowpass filter
      mask Help: helpview(mapfilelocation('dsp'), 'dsplowpassfilter');
      mask Display: disp('Lowpass')
  Mux1 : Mux  Inputs=2
  Scope : Scope
      settings: SaveName=ScopeData8
  Unary Minus : UnaryMinus
  Zero-Order Hold : ZeroOrderHold  SampleTime=.001
  T_lim : Outport
  wires:
  Derivative/1 -> Mux1/1
  Mux1/1 -> Fuzzy Logic  Controller  with Ruleviewer/1
  Fuzzy Logic  Controller  with Ruleviewer/1 -> Scope/1, T_lim/1
  Slip Ratio [%]/1 -> Zero-Order Hold/1
  Abs/1 -> Unary Minus/1
  Unary Minus/1 -> Mux1/2
  Lowpass Filter/1(Out) -> Derivative/1, Abs/1
  Zero-Order Hold/1 -> Lowpass Filter/1(In)

== system AWD_Test_ABS_PID/ABS/AY Control/FR Slip Controller ==
  Slip Ratio [%] : Inport
  Abs : Abs
  Derivative : Derivative
  Fuzzy Logic  Controller  with Ruleviewer : fuzblock/Fuzzy Logic  Controller  with Ruleviewer  SystemSampleTime=-1  fismatrix=Fuzzy_Slip_Controller  Ts=.1
  Mux1 : Mux  Inputs=2
  Scope : Scope
      settings: SaveName=ScopeData8
  Unary Minus : UnaryMinus
  T_lim : Outport
  wires:
  Derivative/1 -> Mux1/1
  Mux1/1 -> Fuzzy Logic  Controller  with Ruleviewer/1
  Fuzzy Logic  Controller  with Ruleviewer/1 -> Scope/1, T_lim/1
  Abs/1 -> Unary Minus/1
  Unary Minus/1 -> Mux1/2
  Slip Ratio [%]/1 -> Derivative/1, Abs/1

== system AWD_Test_ABS_PID/ABS/AY Control/RL Slip Controller ==
  Slip Ratio [%] : Inport
  Abs : Abs
  Derivative : Derivative
  Fuzzy Logic  Controller  with Ruleviewer : fuzblock/Fuzzy Logic  Controller  with Ruleviewer  SystemSampleTime=-1  fismatrix=Fuzzy_Slip_Controller  Ts=.1
  Fuzzy Logic  Controller  with Ruleviewer1 : fuzblock/Fuzzy Logic  Controller  with Ruleviewer  SystemSampleTime=-1  fismatrix=Fuzzy_Slip_Controller  Ts=.1
  Mux1 : Mux  Inputs=2
  Mux2 : Mux  Inputs=2
  Scope : Scope
      settings: SaveName=ScopeData8
  Scope1 : Scope  NumInputPorts=3
      settings: YMin=-5~-5~-5  YMax=5~5~5  SaveName=ScopeData13
  Sine Wave : Sin  Frequency=10  Phase=90  SampleTime=.01
  Sine Wave1 : Sin  Amplitude=.4  Bias=-.5  Frequency=12  SampleTime=.01
  Unary Minus : UnaryMinus
  T_lim : Outport
  wires:
  Derivative/1 -> Mux1/1
  Mux1/1 -> Fuzzy Logic  Controller  with Ruleviewer/1
  Fuzzy Logic  Controller  with Ruleviewer/1 -> Scope/1, T_lim/1
  Abs/1 -> Unary Minus/1
  Unary Minus/1 -> Mux1/2
  Slip Ratio [%]/1 -> Derivative/1, Abs/1
  Fuzzy Logic  Controller  with Ruleviewer1/1 -> Scope1/1
  Mux2/1 -> Fuzzy Logic  Controller  with Ruleviewer1/1
  Sine Wave/1 -> Mux2/1, Scope1/2
  Sine Wave1/1 -> Mux2/2, Scope1/3

== system AWD_Test_ABS_PID/ABS/AY Control/RR Slip Controller ==
  Slip Ratio [%] : Inport
  Abs : Abs
  Derivative : Derivative
  Fuzzy Logic  Controller  with Ruleviewer : fuzblock/Fuzzy Logic  Controller  with Ruleviewer  SystemSampleTime=-1  fismatrix=Fuzzy_Slip_Controller  Ts=.01
  Mux1 : Mux  Inputs=2
  Scope : Scope
      settings: SaveName=ScopeData8
  Unary Minus : UnaryMinus
  T_lim : Outport
  wires:
  Derivative/1 -> Mux1/1
  Mux1/1 -> Fuzzy Logic  Controller  with Ruleviewer/1
  Fuzzy Logic  Controller  with Ruleviewer/1 -> Scope/1, T_lim/1
  Abs/1 -> Unary Minus/1
  Unary Minus/1 -> Mux1/2
  Slip Ratio [%]/1 -> Derivative/1, Abs/1

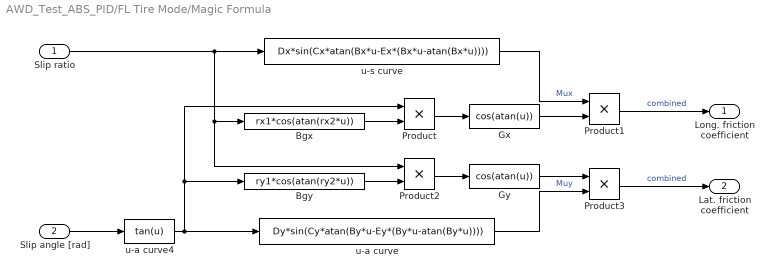
== system AWD_Test_ABS_PID/FL Tire Mode/Magic Formula ==
  Slip ratio : Inport
  Slip angle [rad] : Inport  Port=2
  Bgx : Fcn  Expr=rx1*cos(atan(rx2*u))
  Bgy : Fcn  Expr=ry1*cos(atan(ry2*u))
  Gx : Fcn  Expr=cos(atan(u))
  Gy : Fcn  Expr=cos(atan(u))
  Product{,1..3} (4 alike) : Product  RndMeth=Zero
  u-a curve : Fcn  Expr=Dy*sin(Cy*atan(By*u-Ey*(By*u-atan(By*u))))
  u-a curve4 : Fcn  Expr=tan(u)
  u-s curve : Fcn  Expr=Dx*sin(Cx*atan(Bx*u-Ex*(Bx*u-atan(Bx*u))))
  Long. friction coefficient : Outport
  Lat. friction coefficient : Outport  Port=2
  wires:
  Bgx/1 -> Product/2
  Bgy/1 -> Product2/2
  Slip angle [rad]/1 -> u-a curve4/1
  Product3/1 -> Lat. friction coefficient/1  "combined"
  Gy/1 -> Product3/1
  Product2/1 -> Gy/1
  Product1/1 -> Long. friction coefficient/1  "combined"
  Gx/1 -> Product1/2
  Product/1 -> Gx/1
  u-a curve4/1 -> Product/1, Bgy/1, u-a curve/1
  Slip ratio/1 -> Bgx/1, Product2/1, u-s curve/1
  u-a curve/1 -> Product3/2  "Muy"
  u-s curve/1 -> Product1/1  "Mux"

== system AWD_Test_ABS_PID/FR Tire Mode/Magic Formula ==
  Slip ratio : Inport
  Slip angle [rad] : Inport  Port=2
  Bgx : Fcn  Expr=rx1*cos(atan(rx2*u))
  Bgy : Fcn  Expr=ry1*cos(atan(ry2*u))
  Gx : Fcn  Expr=cos(atan(u))
  Gy : Fcn  Expr=cos(atan(u))
  Product{,1..3} (4 alike) : Product  RndMeth=Zero
  u-a curve : Fcn  Expr=Dy*sin(Cy*atan(By*u-Ey*(By*u-atan(By*u))))
  u-a curve4 : Fcn  Expr=tan(u)
  u-s curve : Fcn  Expr=Dx*sin(Cx*atan(Bx*u-Ex*(Bx*u-atan(Bx*u))))
  Long. firction coefficient : Outport
  Lat. friction coefficient : Outport  Port=2
  wires:
  u-s curve/1 -> Product1/1  "Mux"
  u-a curve/1 -> Product3/2  "Muy"
  Slip ratio/1 -> u-s curve/1, Product2/1, Bgx/1
  u-a curve4/1 -> u-a curve/1, Bgy/1, Product/1
  Product/1 -> Gx/1
  Gx/1 -> Product1/2
  Product1/1 -> Long. firction coefficient/1  "combined"
  Product2/1 -> Gy/1
  Gy/1 -> Product3/1
  Product3/1 -> Lat. friction coefficient/1  "combined"
  Slip angle [rad]/1 -> u-a curve4/1
  Bgy/1 -> Product2/2
  Bgx/1 -> Product/2

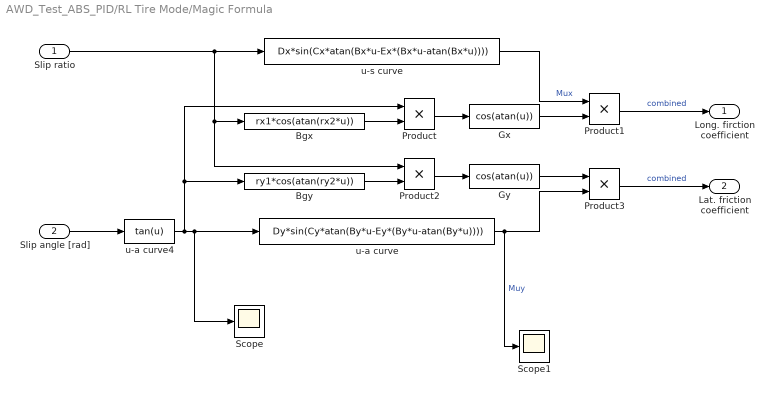
== system AWD_Test_ABS_PID/RL Tire Mode/Magic Formula ==
  Slip ratio : Inport
  Slip angle [rad] : Inport  Port=2
  Bgx : Fcn  Expr=rx1*cos(atan(rx2*u))
  Bgy : Fcn  Expr=ry1*cos(atan(ry2*u))
  Gx : Fcn  Expr=cos(atan(u))
  Gy : Fcn  Expr=cos(atan(u))
  Product{,1..3} (4 alike) : Product  RndMeth=Zero
  Scope : Scope
      settings: TimeRange=21
  Scope1 : Scope
      settings: SaveName=ScopeData4
  u-a curve : Fcn  Expr=Dy*sin(Cy*atan(By*u-Ey*(By*u-atan(By*u))))
  u-a curve4 : Fcn  Expr=tan(u)
  u-s curve : Fcn  Expr=Dx*sin(Cx*atan(Bx*u-Ex*(Bx*u-atan(Bx*u))))
  Long. firction coefficient : Outport
  Lat. friction coefficient : Outport  Port=2
  wires:
  Bgx/1 -> Product/2
  Bgy/1 -> Product2/2
  Slip angle [rad]/1 -> u-a curve4/1
  Product3/1 -> Lat. friction coefficient/1  "combined"
  Gy/1 -> Product3/1
  Product2/1 -> Gy/1
  Product1/1 -> Long. firction coefficient/1  "combined"
  Gx/1 -> Product1/2
  Product/1 -> Gx/1
  u-a curve4/1 -> Product/1, Bgy/1, u-a curve/1, Scope/1
  Slip ratio/1 -> Bgx/1, Product2/1, u-s curve/1
  u-a curve/1 -> Product3/2, Scope1/1  "Muy"
  u-s curve/1 -> Product1/1  "Mux"

== system AWD_Test_ABS_PID/RR Tire Mode/Magic Formula ==
  Slip ratio : Inport
  Slip angle [rad] : Inport  Port=2
  Bgx : Fcn  Expr=rx1*cos(atan(rx2*u))
  Bgy : Fcn  Expr=ry1*cos(atan(ry2*u))
  Gx : Fcn  Expr=cos(atan(u))
  Gy : Fcn  Expr=cos(atan(u))
  Product{,1..3} (4 alike) : Product  RndMeth=Zero
  u-a curve : Fcn  Expr=Dy*sin(Cy*atan(By*u-Ey*(By*u-atan(By*u))))
  u-a curve4 : Fcn  Expr=tan(u)
  u-s curve : Fcn  Expr=Dx*sin(Cx*atan(Bx*u-Ex*(Bx*u-atan(Bx*u))))
  Long. firction coefficient : Outport
  Lat. friction coefficient : Outport  Port=2
  wires:
  u-s curve/1 -> Product1/1  "Mux"
  u-a curve/1 -> Product3/2  "Muy"
  Slip ratio/1 -> u-s curve/1, Product2/1, Bgx/1
  u-a curve4/1 -> u-a curve/1, Bgy/1, Product/1
  Product/1 -> Gx/1
  Gx/1 -> Product1/2
  Product1/1 -> Long. firction coefficient/1  "combined"
  Product2/1 -> Gy/1
  Gy/1 -> Product3/1
  Product3/1 -> Lat. friction coefficient/1  "combined"
  Slip angle [rad]/1 -> u-a curve4/1
  Bgy/1 -> Product2/2
  Bgx/1 -> Product/2

== system AWD_Test_ABS_PID/Wheel States/Subsystem1 ==
  slip angle : Inport
  long. speed [m/s] : Inport  Port=2
  If : If
  Merge1 : Merge
  negative slip angle : Subsystem  TreatAsAtomicUnit=on
  positive slip angle : Subsystem  TreatAsAtomicUnit=on
  slip angle [rad] : Outport
  wires:
  If/2 -> negative slip angle/Action
  negative slip angle/1(-in) -> Merge1/2
  positive slip angle/1(+in) -> Merge1/1
  If/1 -> positive slip angle/Action
  long. speed [m/s]/1 -> If/1
  slip angle/1 -> negative slip angle/1(in), positive slip angle/1(in)
  Merge1/1 -> slip angle [rad]/1

== system AWD_Test_ABS_PID/Wheel States/Subsystem2 ==
  slip angle : Inport
  long. speed [m/s] : Inport  Port=2
  If : If
  Merge1 : Merge
  negative slip angle : Subsystem  TreatAsAtomicUnit=on
  positive slip angle : Subsystem  TreatAsAtomicUnit=on
  slip angle [rad] : Outport
  wires:
  Merge1/1 -> slip angle [rad]/1
  slip angle/1 -> positive slip angle/1(in), negative slip angle/1(in)
  long. speed [m/s]/1 -> If/1
  If/1 -> positive slip angle/Action
  positive slip angle/1(+in) -> Merge1/1
  negative slip angle/1(-in) -> Merge1/2
  If/2 -> negative slip angle/Action

== system AWD_Test_ABS_PID/Wheel States/Subsystem3 ==
  slip angle : Inport
  long. speed [m/s] : Inport  Port=2
  If : If
  Merge1 : Merge
  negative slip angle : Subsystem  TreatAsAtomicUnit=on
  positive slip angle : Subsystem  TreatAsAtomicUnit=on
  slip angle [rad] : Outport
  wires:
  Merge1/1 -> slip angle [rad]/1
  slip angle/1 -> positive slip angle/1(in), negative slip angle/1(in)
  long. speed [m/s]/1 -> If/1
  If/1 -> positive slip angle/Action
  positive slip angle/1(+in) -> Merge1/1
  negative slip angle/1(-in) -> Merge1/2
  If/2 -> negative slip angle/Action

== system AWD_Test_ABS_PID/Wheel States/Subsystem4 ==
  slip angle : Inport
  long. speed [m/s] : Inport  Port=2
  If : If
  Merge1 : Merge
  negative slip angle : Subsystem  TreatAsAtomicUnit=on
  positive slip angle : Subsystem  TreatAsAtomicUnit=on
  slip angle [rad] : Outport
  wires:
  If/2 -> negative slip angle/Action
  negative slip angle/1(-in) -> Merge1/2
  positive slip angle/1(+in) -> Merge1/1
  If/1 -> positive slip angle/Action
  long. speed [m/s]/1 -> If/1
  slip angle/1 -> negative slip angle/1(in), positive slip angle/1(in)
  Merge1/1 -> slip angle [rad]/1

== system AWD_Test_ABS_PID/ABS/AY Control/FL Slip Controller/Lowpass Filter ==
  In : Inport
  Generated Filter Block : dsparch4/Digital Filter  Tag=BlockMethodSubSystem  TypePopup=FIR (all zeros)  IIRFiltStruct=Direct form II transposed  AllPoleFiltStruct=Direct form  FIRFiltStruct=Direct form  CoeffSource=Specify via dialog  NumCoeffs=[0.0174383341854297 -0.00191782029741124 0.00198412368845642 -0.00202320724480635 0.00203368000831878 -0.00201284299964119 0.0019583382808233 -0.00186738997518325 0.00173746587339042 -0.0015681629128845 0.00135498370854467 -0.00110302068622745 0.000800701191448522 -0.000457496942976669 6.66695446854202e-005 0.000372926543227212 -0.000859609238705387 0.00139275199781003 -0.00197359205968968 0.00260213773222492 -0.00327367392723359 0.00399185205153304 -0.00474687033612613 0.00553984252048373 -0.00636388746973452 0.00721789141475684 -0.00809980835965676 0.00900839900993329 -0.00994311352927216 0.0109001841792156 -0.0118658172469424 0.0127965798493482 -0.0137852818010553 0.014742027667021 -0.0156964264578652 0.0166370406414232 -0.0175588861083261 0.0184562272582075 -0.0193239272144743 0.0201573063619979 -0.0209504538297715 0.0217022550324855 -0.0223968347980343 0.0230523485789057 -0.023639833722988 0.0241679591776366 -0.0246360803373166 0.025038665505458 -0.0253705205926199 0.0256294834812449 -0.0258148349606314 0.0259242151526749 0.974037626336816 0.0259242151526749 -0.0258148349606314 0.0256294834812449 -0.0253705205926199 0.025038665505458 -0.0246360803373166 0.0241679591776366 -0.023639833722988 0.0230523485789057 -0.0223968347980343 0.0217022550324855 -0.0209504538297715 0.0201573063619979 -0.0193239272144743 0.0184562272582075 -0.0175588861083261 0.0166370406414232 -0.0156964264578652 0.014742027667021 -0.0137852818010553 0.0127965798493482 -0.0118658172469424 0.0109001841792156 -0.00994311352927216 0.00900839900993329 -0.00809980835965676 0.00721789141475684 -0.00636388746973452 0.00553984252048373 -0.00474687033612613 0.00399185205153304 -0.00327367392723359 0.00260213773222492 -0.00197359205968968 0.00139275199781003 -0.000859609238705387 0.000372926543227212 6.66695446854202e-005 -0.000457496942976669 0.000800701191448522 -0.00110302068622745 0.00135498370854467 -0.0015681629128845 0.00173746587339042 -0.00186738997518325 0.0019583382808233 -0.00201284299964119 0.00203368000831878 -0.00202320724480635 0.00198412368845642 -0.00191782029741124 0.0174383341854297]  DenCoeffs=[1 0.1]  BiQuadCoeffs=[1 0.3 0.4 1 0.1 0.2]  LatticeCoeffs=[0.2 0.4]  denIgnore=on  FiltPerSampPopup=One filter per frame  IC=0  ICnum=0  ICden=0  roundingMode=Floor  overflowMode=off  ScaleValues=1  scaleValueFracLength=14  stageInFracLength=15  stageOutFracLength=15  FilterSource=Specify via dialog  dfiltObjectName=dfilt.dffir([1 2 1])  InputProcessing=Columns as channels (frame based)
  Out : Outport
  wires:
  In/1 -> Generated Filter Block/1
  Generated Filter Block/1 -> Out/1

== system AWD_Test_ABS_PID/Wheel States/Subsystem1/negative slip angle ==
  in : Inport
  Action Port : ActionPort  ActionType=else
  Gain : Gain  Gain=-1
  -in : Outport
  wires:
  in/1 -> Gain/1
  Gain/1 -> -in/1

== system AWD_Test_ABS_PID/Wheel States/Subsystem1/positive slip angle ==
  in : Inport
  Action Port : ActionPort  ActionType=then
  +in : Outport
  wires:
  in/1 -> +in/1

== system AWD_Test_ABS_PID/Wheel States/Subsystem2/negative slip angle ==
  in : Inport
  Action Port : ActionPort  ActionType=else
  Gain : Gain  Gain=-1
  -in : Outport
  wires:
  Gain/1 -> -in/1
  in/1 -> Gain/1

== system AWD_Test_ABS_PID/Wheel States/Subsystem2/positive slip angle ==
  in : Inport
  Action Port : ActionPort  ActionType=then
  +in : Outport
  wires:
  in/1 -> +in/1

== system AWD_Test_ABS_PID/Wheel States/Subsystem3/negative slip angle ==
  in : Inport
  Action Port : ActionPort  ActionType=else
  Gain : Gain  Gain=-1
  -in : Outport
  wires:
  Gain/1 -> -in/1
  in/1 -> Gain/1

== system AWD_Test_ABS_PID/Wheel States/Subsystem3/positive slip angle ==
  in : Inport
  Action Port : ActionPort  ActionType=then
  +in : Outport
  wires:
  in/1 -> +in/1

== system AWD_Test_ABS_PID/Wheel States/Subsystem4/negative slip angle ==
  in : Inport
  Action Port : ActionPort  ActionType=else
  Gain : Gain  Gain=-1
  -in : Outport
  wires:
  in/1 -> Gain/1
  Gain/1 -> -in/1

== system AWD_Test_ABS_PID/Wheel States/Subsystem4/positive slip angle ==
  in : Inport
  Action Port : ActionPort  ActionType=then
  +in : Outport
  wires:
  in/1 -> +in/1
